simulink model "regulatory"  (R2024b)
settings: Solver=ode45  StartTime=0.0  StopTime=10.0  RelTol=1e-3
settings Model: Creator=juliawilkosz  LastModifiedBy=juliawilkosz

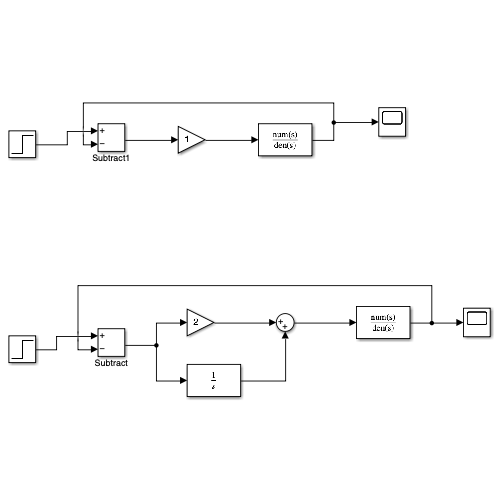
[thumbnail: Simulink's stored preview of the top-level diagram]
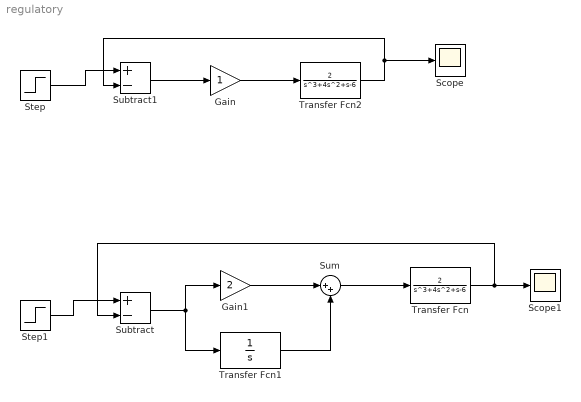
== system regulatory ==
  Gain : Gain
  Gain1 : Gain  Gain=2
  Scope : Scope
  Scope1 : Scope
  Step : Step  SampleTime=0
  Step1 : Step  SampleTime=0
  Subtract : Sum  Inputs=+-
  Subtract1 : Sum  Inputs=+-
  Sum : Sum  Inputs=|++
  Transfer Fcn : TransferFcn  Numerator=[2]  Denominator=[1 4 1 -6]
  Transfer Fcn1 : TransferFcn  Denominator=[1 0]
  Transfer Fcn2 : TransferFcn  Numerator=[2]  Denominator=[1 4 1 -6]
  wires:
  Gain1/1 -> Sum/1
  Transfer Fcn1/1 -> Sum/2
  Sum/1 -> Transfer Fcn/1
  Step1/1 -> Subtract/1
  Transfer Fcn/1 -> Subtract/2, Scope1/1
  Subtract/1 -> Transfer Fcn1/1, Gain1/1
  Step/1 -> Subtract1/1
  Subtract1/1 -> Gain/1
  Gain/1 -> Transfer Fcn2/1
  Transfer Fcn2/1 -> Scope/1, Subtract1/2
